simulink model "OneFour_2_block"  (R2022b)
settings: Solver=VariableStepAuto  StartTime=0.0  StopTime=10  MaxStep=1e-3  MinStep=1e-4  RelTol=1e-3
libraries: simulink x1
settings Model: Creator=yeyi5  LastModifiedBy=yeyi5

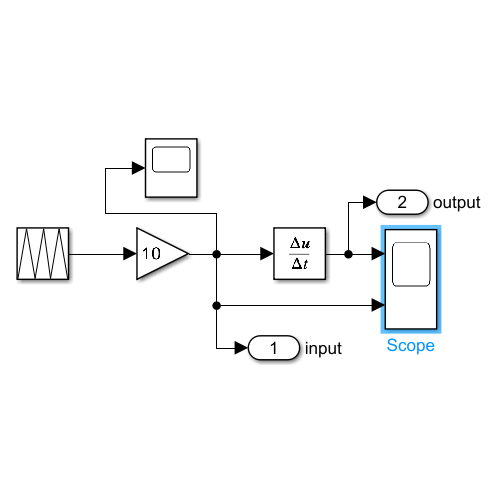
[thumbnail: Simulink's stored preview of the top-level diagram]
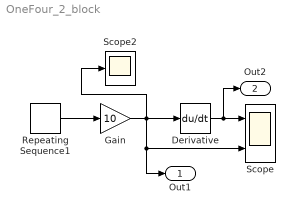
== system OneFour_2_block ==
  Derivative : Derivative
  Gain : Gain  Gain=10
  Repeating Sequence1 : simulink/Sources/Repeating Sequence  rep_seq_t=[0, 0.5/0.5, 1/0.5]  rep_seq_y=[-1, 1, -1]
  Scope : Scope  NumInputPorts=2
  Scope2 : Scope
  Out1 : Outport  SignalName=input
  Out2 : Outport  Port=2  SignalName=output
  wires:
  Repeating Sequence1/1 -> Gain/1
  Gain/1 -> Out1/1, Scope/2, Scope2/1, Derivative/1
  Derivative/1 -> Out2/1, Scope/1
